simulink model "test10"  (R2021a)
settings: Solver=VariableStepAuto  StartTime=0.0  StopTime=8  RelTol=1e-3
model workspace (MAT data in the model file):
  params = climate_p
libraries: HORTISIM x5
settings Model: SimulationMode=accelerator  Creator=djoroya  LastModifiedBy=djoroya
settings DebuggingCC: UnconnectedInputMsg=none  UnconnectedOutputMsg=none  UnconnectedLineMsg=none

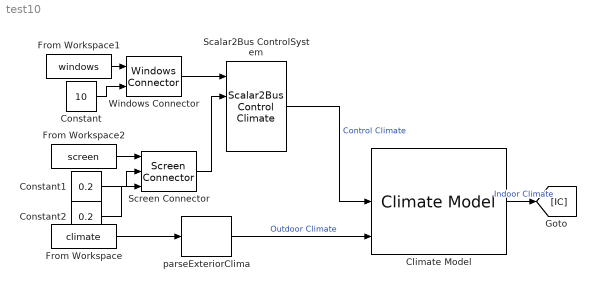
== system test10 ==
  Climate Model : HORTISIM/Climate/Models/Climate Model  params=params  x0=cic
      settings: SourceProductName=Horti Simulator
  Constant : Constant  Value=10
  Constant1 : Constant  Value=0.2
  Constant2 : Constant  Value=0.2
  From Workspace : FromWorkspace  VariableName=climate
  From Workspace1 : FromWorkspace  VariableName=windows
  From Workspace2 : FromWorkspace  VariableName=screen
  Scalar2Bus ControlSystem : HORTISIM/Other  Functions/Scalar2Bus  Control Climate  SystemSampleTime=-1  VariantActivationTime=update diagram  Latency=0  AutoFrameSizeCalculation=off
      settings: SourceProductName=Horti Simulator
  Screen Connector : HORTISIM/Other  Functions/Screen Connector  SystemSampleTime=-1  VariantActivationTime=update diagram  Latency=0  AutoFrameSizeCalculation=off
      settings: SourceProductName=Horti Simulator
  Windows Connector : HORTISIM/Other  Functions/Windows Connector  SystemSampleTime=-1  VariantActivationTime=update diagram  Latency=0  AutoFrameSizeCalculation=off
      settings: SourceProductName=Horti Simulator
  parseExteriorClima : HORTISIM/Other  Functions/parseExteriorClima  SystemSampleTime=-1  VariantActivationTime=update diagram  Latency=0  AutoFrameSizeCalculation=off
      settings: SourceProductName=Horti Simulator
  wires:
  From Workspace/1 -> parseExteriorClima/1
  parseExteriorClima/1 -> Climate Model/3  "Outdoor Climate"
  Climate Model/1 -> [IC]  "Indoor Climate"
  Scalar2Bus ControlSystem/1 -> Climate Model/2  "Control Climate"
  Windows Connector/1 -> Scalar2Bus ControlSystem/1
  From Workspace1/1 -> Windows Connector/1
  Constant/1 -> Windows Connector/2
  From Workspace2/1 -> Screen Connector/1
  Constant1/1 -> Screen Connector/2
  Constant2/1 -> Screen Connector/3
  Screen Connector/1 -> Scalar2Bus ControlSystem/2
